simulink model "msd_system"  (Simulink 6.0)
settings: Solver=ode3  StartTime=0  StopTime=4  FixedStep=0.1  RelTol=1e-3
model workspace (MAT data in the model file):
  F = 100
  m = 8
  b = 100
  k : num (value not decoded)
PreLoadFcn:
  | load msd_system
settings Model: Creator=beryilma  LastModifiedBy=rsingh
settings DataIOCC: LimitDataPoints=off  SaveOutput=off  SaveTime=off  SignalLoggingName=logsOut
settings DebuggingCC: CheckExecutionContextPreStartOutputMsg=on  CheckExecutionContextRuntimeOutputMsg=on  SolverPrmCheckMsg=none
settings SFSimCC: SFSimApplyToAllLibs=on  SFSimBuildMode=Incremental

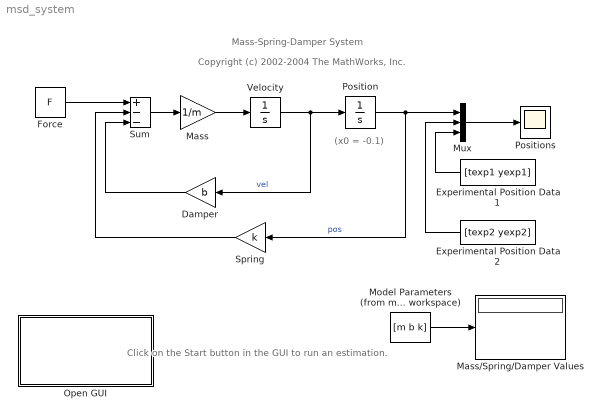
== system msd_system ==
  note: Click on the Start button in the GUI
      | to run an estimation.
  note: Mass-Spring-Damper System
  note: Copyright (c) 2002-2004 The MathWorks, Inc.
  note: (x0 = -0.1)
  Damper : Gain  Orientation=left  Gain=b  SaturateOnIntegerOverflow=on
  Experimental Position Data 1 : FromWorkspace  Orientation=left  VariableName=[texp1 yexp1]  SampleTime=0  OutputAfterFinalValue=Holding final value
  Experimental Position Data 2 : FromWorkspace  Orientation=left  VariableName=[texp2 yexp2]  SampleTime=0  OutputAfterFinalValue=Holding final value
  Force : Constant  Value=F
  Mass : Gain  Gain=1/m  SaturateOnIntegerOverflow=on
  Mass/Spring/Damper Values : Display
  Model Parameters (from model workspace) : Constant  Value=[m b k]
  Mux : Mux  Inputs=3
  Open GUI : Subsystem  PropExecContextAcrossSSBoundary=on
      settings: OpenFcn=|
      | [F,W,M] = slctrlexplorer('initialize');
      | p = M.load('msd_system_project');
      | W.addNode(p);
      | h = find(p, '-class', 'spenodes.EstimationLeaf');
      | F.setSelected(h(1).getTreeNodeInterface);
      | drawnow;
      | runpanel = h(1).getDialogInterface(M).getEstimationRun;  tabpanel = runpanel.getParent; awtinvoke(tabpanel, 'setSelectedComponent', runpanel);
      | F.setVisible(1);
      mask Display: disp('Double click here\nto open the\nParameter Estimation\nGUI with preloaded data')
  Position : Integrator  InitialCondition=-0.1
  Positions : Scope
      settings: TimeRange=4  YMin=-0.1  YMax=0.3
  Spring : Gain  Orientation=left  Gain=k  SaturateOnIntegerOverflow=on
  Sum : Sum  Inputs=+--  SaturateOnIntegerOverflow=on  InputSameDT=on
  Velocity : Integrator
  wires:
  Velocity/1 -> Position/1, Damper/1  "vel"
  Position/1 -> Spring/1, Mux/1  "pos"
  Sum/1 -> Mass/1
  Damper/1 -> Sum/3
  Spring/1 -> Sum/2
  Force/1 -> Sum/1
  Mass/1 -> Velocity/1
  Model Parameters (from model workspace)/1 -> Mass/Spring/Damper Values/1
  Mux/1 -> Positions/1
  Experimental Position Data 1/1 -> Mux/3
  Experimental Position Data 2/1 -> Mux/2

== system msd_system/Open GUI ==
